simulink model "SIGAS_Controller"  (R2026a)
settings: Solver=FixedStepDiscrete  StopTime=Test_DefaultStopTime  FixedStep=Timing_PressureSample
undefined symbols (not defined in the file): GasSensor_High, GasSensor_WarningEnter, GasSensor_WarningExit, Pressure_Delta, Pressure_Low, Pressure_SupplyLow, Timing_GasSample, Timing_PressureSample
settings Model: DataDictionary=sigas_rt.sldd  Creator=josue  LastModifiedBy=josue

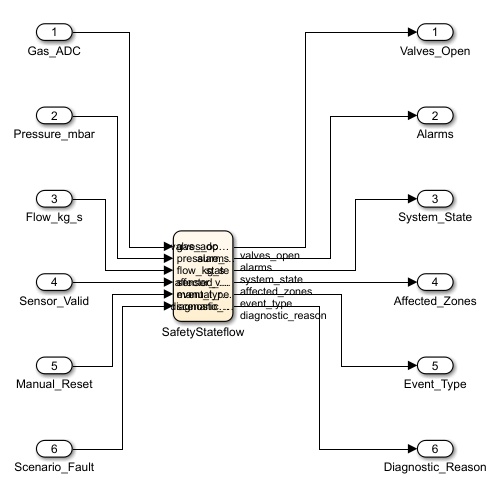
[thumbnail: Simulink's stored preview of the top-level diagram]
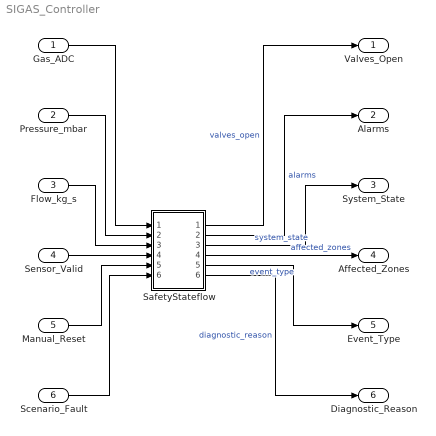
== system SIGAS_Controller ==
  Gas_ADC : Inport  OutDataTypeStr=uint16  PortDimensions=3  SampleTime=0.05
  Pressure_mbar : Inport  Port=2  OutDataTypeStr=double  PortDimensions=5  SampleTime=0.05
  Flow_kg_s : Inport  Port=3  OutDataTypeStr=double  PortDimensions=2  SampleTime=0.05
  Sensor_Valid : Inport  Port=4  OutDataTypeStr=boolean  PortDimensions=3  SampleTime=0.05
  Manual_Reset : Inport  Port=5  OutDataTypeStr=boolean  PortDimensions=1  SampleTime=0.05
  Scenario_Fault : Inport  Port=6  OutDataTypeStr=boolean  PortDimensions=1  SampleTime=0.05
  SafetyStateflow : Stateflow chart  TreatAsAtomicUnit=on
  Valves_Open : Outport
  Alarms : Outport  Port=2
  System_State : Outport  Port=3
  Affected_Zones : Outport  Port=4
  Event_Type : Outport  Port=5
  Diagnostic_Reason : Outport  Port=6
  wires:
  SafetyStateflow/6(diagnostic_reason) -> Diagnostic_Reason/1  "diagnostic_reason"
  SafetyStateflow/5(event_type) -> Event_Type/1  "event_type"
  SafetyStateflow/4(affected_zones) -> Affected_Zones/1  "affected_zones"
  SafetyStateflow/3(state) -> System_State/1  "system_state"
  SafetyStateflow/2(alarms) -> Alarms/1  "alarms"
  SafetyStateflow/1(valves_open) -> Valves_Open/1  "valves_open"
  Scenario_Fault/1 -> SafetyStateflow/6(scenario_fault)
  Manual_Reset/1 -> SafetyStateflow/5(manual_reset)
  Sensor_Valid/1 -> SafetyStateflow/4(sensor_valid)
  Flow_kg_s/1 -> SafetyStateflow/3(flow_kg_s)
  Pressure_mbar/1 -> SafetyStateflow/2(pressure_mbar)
  Gas_ADC/1 -> SafetyStateflow/1(gas_adc)

== stateflow chart SIGAS_Controller/SafetyStateflow ==
  state STARTUP
    en: state=uint8(0); valves_open=[false;false;false;false]; alarms=[false;false;true]; latched_event=uint8(0); latched_zones=uint8(0); affected_zones=latched_zones; event_type=latched_event; diagnostic_reason=uint8(0);
  state NORMAL
    en: state=uint8(1); valves_open=[true;true;true;true]; alarms=[false;true;false]; latched_event=uint8(0); latched_zones=uint8(0); affected_zones=latched_zones; event_type=latched_event; diagnostic_reason=uint8(0);
  state WARNING
    en: state=uint8(2); valves_open=[true;true;true;true]; alarms=[false;true;true]; latched_event=uint8(0); latched_zones=uint8(0); affected_zones=latched_zones; event_type=latched_event; diagnostic_reason=uint8(1);
  state CRITICAL
    en: state=uint8(3); alarms=[true;false;true]; event_type=latched_event; affected_zones=latched_zones; diagnostic_reason=uint8(3); if latched_event==uint8(5) || latched_event==uint8(6), valves_open=[false;false;false;false]; else, valves_open=[true; bitand(latched_zones,uint8(1))==0; bitand(latched_zones,uint8(2))==0; bitand(latched_zones,uint8(4))==0]; end
  state SAFE_LATCHED
    en: state=uint8(4); alarms=[true;false;true]; event_type=latched_event; affected_zones=latched_zones; diagnostic_reason=uint8(3); if latched_event==uint8(5) || latched_event==uint8(6), valves_open=[false;false;false;false]; else, valves_open=[true; bitand(latched_zones,uint8(1))==0; bitand(latched_zones,uint8(2))==0; bitand(latched_zones,uint8(4))==0]; end
  state FAULT
    en: state=uint8(5); valves_open=[false;false;false;false]; alarms=[true;false;true]; latched_event=uint8(4); latched_zones=uint8(0); affected_zones=latched_zones; event_type=latched_event; diagnostic_reason=uint8(2);
  (default) -> STARTUP
  STARTUP -> NORMAL [order 2] : [duration(all(sensor_valid) && all(gas_adc < GasSensor_WarningExit)) >= (2*Timing_GasSample)]
  STARTUP -> FAULT [order 1] : [scenario_fault || ~all(sensor_valid)]
  FAULT -> STARTUP : [manual_reset && ~scenario_fault && duration(all(sensor_valid) && all(gas_adc < GasSensor_WarningExit) && pressure_mbar(1) >= Pressure_Low && all(pressure_mbar(3:5) >= Pressure_Low)) >= (2*Timing_GasSample)]
  SAFE_LATCHED -> STARTUP [order 2] : [manual_reset && duration(all(sensor_valid) && all(gas_adc < GasSensor_WarningExit) && pressure_mbar(1) >= Pressure_Low && all(pressure_mbar(3:5) >= Pressure_Low)) >= (2*Timing_GasSample)]
  NORMAL -> FAULT [order 1] : [scenario_fault || ~all(sensor_valid)]
  WARNING -> NORMAL [order 9] : [all(gas_adc < GasSensor_WarningExit) && pressure_mbar(1) >= Pressure_Low && all(pressure_mbar(3:5) >= Pressure_Low)]
  NORMAL -> WARNING [order 2] : [any(gas_adc >= GasSensor_WarningEnter) || pressure_mbar(1) < Pressure_SupplyLow || (pressure_mbar(2) >= Pressure_Low && any(pressure_mbar(3:5) < Pressure_Low))]
  WARNING -> FAULT [order 1] : [scenario_fault || ~all(sensor_valid)]
  WARNING -> CRITICAL [order 2] : [duration(sum(gas_adc >= GasSensor_High) >= 2) >= (2*Timing_GasSample)]/{latched_event=uint8(5); latched_zones=uint8(7);}
  WARNING -> CRITICAL [order 3] : [duration(pressure_mbar(1) < Pressure_SupplyLow && all(pressure_mbar(2:5) < Pressure_Low)) >= (2*Timing_PressureSample)]/{latched_event=uint8(6); latched_zones=uint8(7);}
  WARNING -> CRITICAL [order 4] : [duration(pressure_mbar(2) >= Pressure_Low && pressure_mbar(5) < Pressure_Low && (pressure_mbar(2)-pressure_mbar(5)) >= Pressure_Delta && flow_kg_s(2) > 0 && gas_adc(3) >= GasSensor_High) >= (2*Timing_GasSample)]/{latched_event=uint8(3); latched_zones=uint8(4);}
  WARNING -> CRITICAL [order 5] : [duration(gas_adc(1) >= GasSensor_High) >= (2*Timing_GasSample)]/{latched_event=uint8(1); latched_zones=uint8(1);}
  WARNING -> CRITICAL [order 6] : [duration(gas_adc(2) >= GasSensor_High) >= (2*Timing_GasSample)]/{latched_event=uint8(1); latched_zones=uint8(2);}
  WARNING -> CRITICAL [order 7] : [duration(gas_adc(3) >= GasSensor_High) >= (2*Timing_GasSample)]/{latched_event=uint8(1); latched_zones=uint8(4);}
  WARNING -> CRITICAL [order 8] : [duration(pressure_mbar(2) >= Pressure_Low && any(pressure_mbar(3:5) < Pressure_Low)) >= (20*Timing_PressureSample)]/{latched_event=uint8(2); latched_zones=uint8(0);}
  CRITICAL -> SAFE_LATCHED : [after(1,tick)]
  SAFE_LATCHED -> FAULT [order 1] : [scenario_fault || ~all(sensor_valid)]
  data: gas_adc input uint16; pressure_mbar input double; flow_kg_s input double; sensor_valid input boolean; manual_reset input boolean; scenario_fault input boolean; valves_open output boolean; alarms output boolean; state output uint8; affected_zones output uint8; event_type output uint8; diagnostic_reason output uint8; GasSensor_WarningEnter parameter uint16; GasSensor_WarningExit parameter uint16; GasSensor_High parameter uint16; Pressure_Low parameter double; Pressure_SupplyLow parameter double; Pressure_Delta parameter double; Timing_GasSample parameter double; Timing_PressureSample parameter double; latched_event local uint8; latched_zones local uint8
